simulink model "System_Observer"  (R2016a)
settings: Solver=VariableStepAuto  StartTime=0.0  StopTime=30  RelTol=1e-3
undefined symbols (not defined in the file or in its folder): A_dz, B_dz, C_dz, L
settings Model: Creator=Loki  LastModifiedBy=Loki
settings DataIOCC: LimitDataPoints=on
settings DebuggingCC: AllowSymbolicDim=off
settings ModelReferenceCC: PropagateSignalLabelsOutOfModel=off
settings GRTTargetCC: GeneratePreprocessorConditionals=Use local settings

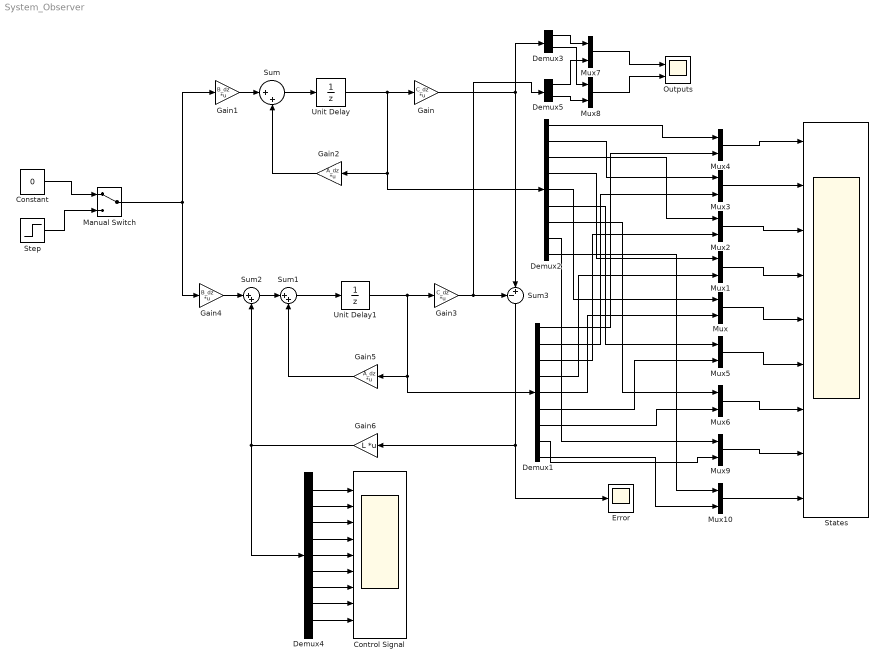
== system System_Observer ==
  Constant : Constant  Value=0  SampleTime=0.001
  Control Signal : Scope  NumInputPorts=9
  Demux1 : Demux  Outputs=9
  Demux2 : Demux  Outputs=9
  Demux3 : Demux  Outputs=2
  Demux4 : Demux  Outputs=9
  Demux5 : Demux  Outputs=2
  Error : Scope
  Gain : Gain  Gain=C_dz  Multiplication=Matrix(K*u)
  Gain1 : Gain  Gain=B_dz  Multiplication=Matrix(K*u)
  Gain2 : Gain  Gain=A_dz  Multiplication=Matrix(K*u)
  Gain3 : Gain  Gain=C_dz  Multiplication=Matrix(K*u)
  Gain4 : Gain  Gain=B_dz  Multiplication=Matrix(K*u)
  Gain5 : Gain  Gain=A_dz  Multiplication=Matrix(K*u)
  Gain6 : Gain  Gain=L  Multiplication=Matrix(K*u)
  Manual Switch : ManualSwitch
  Mux{,1..10} (11 alike) : Mux  Inputs=2
  Outputs : Scope  NumInputPorts=2
  States : Scope  NumInputPorts=9
  Step : Step  SampleTime=0.001
  Sum : Sum  Inputs=|++
  Sum1 : Sum  Inputs=|++
  Sum2 : Sum  Inputs=|++
  Sum3 : Sum  Inputs=-+|
  Unit Delay : UnitDelay  InitialCondition=0.01  SampleTime=0.001
  Unit Delay1 : UnitDelay  SampleTime=0.001
  wires:
  Unit Delay/1 -> Demux2/1, Gain2/1, Gain/1
  Sum/1 -> Unit Delay/1
  Unit Delay1/1 -> Demux1/1, Gain5/1, Gain3/1
  Sum1/1 -> Unit Delay1/1
  Gain5/1 -> Sum1/2
  Manual Switch/1 -> Gain1/1, Gain4/1
  Gain4/1 -> Sum2/1
  Sum2/1 -> Sum1/1
  Gain/1 -> Sum3/2, Demux3/1
  Sum3/1 -> Error/1, Gain6/1
  Gain6/1 -> Sum2/2, Demux4/1
  Demux2/2 -> Mux3/1
  Demux2/4 -> Mux1/1
  Demux1/2 -> Mux3/2
  Demux1/4 -> Mux1/2
  Demux2/5 -> Mux/1
  Demux1/5 -> Mux/2
  Demux2/1 -> Mux4/1
  Demux1/1 -> Mux4/2
  Demux1/3 -> Mux2/2
  Demux2/3 -> Mux2/1
  Gain3/1 -> Sum3/1, Demux5/1
  Mux7/1 -> Outputs/1
  Demux3/1 -> Mux7/1
  Demux5/1 -> Mux7/2
  Demux3/2 -> Mux8/1
  Mux8/1 -> Outputs/2
  Demux5/2 -> Mux8/2
  Constant/1 -> Manual Switch/1
  Step/1 -> Manual Switch/2
  Gain2/1 -> Sum/2
  Gain1/1 -> Sum/1
  Mux4/1 -> States/1
  Mux3/1 -> States/2
  Mux2/1 -> States/3
  Mux1/1 -> States/4
  Mux/1 -> States/5
  Mux5/1 -> States/6
  Mux6/1 -> States/7
  Mux9/1 -> States/8
  Mux10/1 -> States/9
  Demux2/9 -> Mux10/1
  Demux1/9 -> Mux10/2
  Demux2/6 -> Mux5/1
  Demux1/6 -> Mux5/2
  Demux2/7 -> Mux6/1
  Demux1/7 -> Mux6/2
  Demux2/8 -> Mux9/1
  Demux1/8 -> Mux9/2
  Demux4/1 -> Control Signal/1
  Demux4/2 -> Control Signal/2
  Demux4/3 -> Control Signal/3
  Demux4/4 -> Control Signal/4
  Demux4/5 -> Control Signal/5
  Demux4/6 -> Control Signal/6
  Demux4/7 -> Control Signal/7
  Demux4/8 -> Control Signal/8
  Demux4/9 -> Control Signal/9
